simulink model "modelul2cerinta14"  (R2022b)
settings: Solver=VariableStepAuto  StartTime=0.0  StopTime=30  RelTol=1e-3
values from neighbouring files (symbols this model uses):
  SysLinD = c2d(SysLin,Te,'tustin')    [NeleptcuDanielAndrei.m]
  Te = 0.1    [NeleptcuDanielAndrei.m]
undefined symbols (not defined in the file or in its folder): par, ustar8, ystar8
settings Model: Creator=zuch3e  LastModifiedBy=zuch3e
settings DataIOCC: ReturnWorkspaceOutputs=off

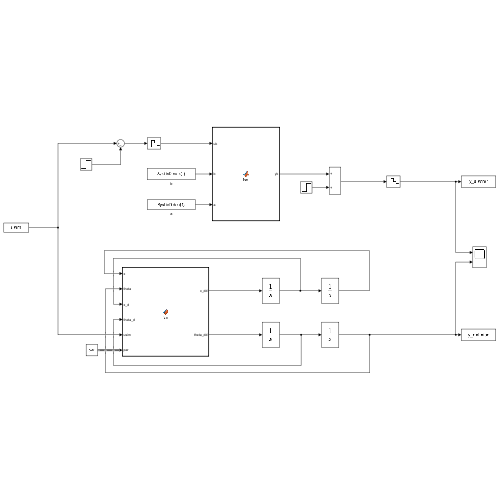
[thumbnail: Simulink's stored preview of the top-level diagram]
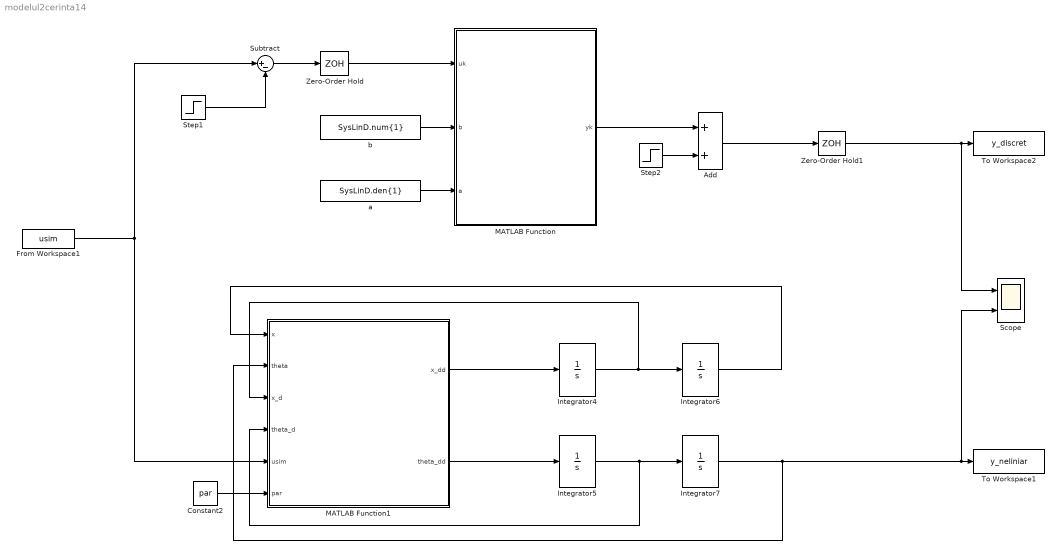
== system modelul2cerinta14 ==
  Add : Sum
  Constant2 : Constant  Value=par  OutDataTypeStr=Bus: par_bus
  From Workspace1 : FromWorkspace  VariableName=usim
  Integrator{4..7} (4 alike) : Integrator
  MATLAB Function : MATLAB Function  TreatAsAtomicUnit=on
  MATLAB Function1 : MATLAB Function  TreatAsAtomicUnit=on
  Scope : Scope  NumInputPorts=2
  Step1 : Step  After=ustar8  SampleTime=0
  Step2 : Step  After=ystar8  SampleTime=0
  Subtract : Sum  Inputs=|+-
  To Workspace1 : ToWorkspace  VariableName=y_neliniar  SaveFormat=Timeseries  SampleTime=-1
  To Workspace2 : ToWorkspace  VariableName=y_discret  SaveFormat=Timeseries  SampleTime=-1
  Zero-Order Hold : ZeroOrderHold  SampleTime=Te
  Zero-Order Hold1 : ZeroOrderHold  SampleTime=Te
  a : Constant  Value=SysLinD.den{1}
  b : Constant  Value=SysLinD.num{1}
  wires:
  Subtract/1 -> Zero-Order Hold/1
  Zero-Order Hold/1 -> MATLAB Function/1(uk)
  Add/1 -> Zero-Order Hold1/1
  Step1/1 -> Subtract/2
  Step2/1 -> Add/2
  From Workspace1/1 -> Subtract/1, MATLAB Function1/5(usim)
  b/1 -> MATLAB Function/2(b)
  a/1 -> MATLAB Function/3(a)
  Integrator4/1 -> MATLAB Function1/3(x_d), Integrator6/1
  Constant2/1 -> MATLAB Function1/6(par)
  Integrator5/1 -> MATLAB Function1/4(theta_d), Integrator7/1
  Integrator6/1 -> MATLAB Function1/1(x)
  MATLAB Function1/2(theta_dd) -> Integrator5/1
  Integrator7/1 -> MATLAB Function1/2(theta), Scope/2, To Workspace1/1
  MATLAB Function1/1(x_dd) -> Integrator4/1
  MATLAB Function/1(yk) -> Add/1
  Zero-Order Hold1/1 -> Scope/1, To Workspace2/1

== matlab function modelul2cerinta14/MATLAB Function1 ==
  data: x input; x_dd output; theta input; x_d input; theta_d input; usim input; par input; theta_dd output
function [x_dd, theta_dd] = fcn(x,theta,x_d,theta_d,usim, par)
x_dd = ((par.l0 + x) * (theta_d^2)) - (par.k*x)/par.m + par.g*cos(theta) - par.zeta*x_d;
theta_dd = ((-1)*par.g*sin(theta))/(par.l0 + x) - (2*x_d*theta_d)/(par.l0 + x) - par.zeta*theta_d + usim/(par.m*((par.l0 + x)^2));
end

== matlab function modelul2cerinta14/MATLAB Function ==
  data: uk input; yk output; b input; a input
function yk = fcn(uk,b,a)

persistent uk1 uk2 uk3 uk4 yk1 yk2 yk3 yk4

% b - coef pt numaratorul functiei de transfer
% a - coef pt numitorul functiei de transfer
[b0,b1,b2,b3,b4,a0,a1,a2,a3,a4] = deal(b(1),b(2),b(3),b(4),b(5),a(1),a(2),a(3),a(4),a(5));


%Verific daca sunt la inceput si nu am nimic in uk si yk
if isempty(uk1) && isempty(uk2) && isempty(uk3) && isempty(uk4) && isempty(yk1) && isempty(yk2) && isempty(yk3) && isempty(yk4)
    [uk1,uk2,uk3,uk4,yk1,yk2,yk3,yk4] = deal(0,0,0,0,0,0,0,0);
end


%Ecuatia cu diferente echivalenta cu cea construita in codul matlab
yk = (1/a0) * (b0*uk + b1*uk1 + b2*uk2 + b3*uk3 + b4*uk4 - a1*yk1 - a2*yk2 - a3*yk3 - a4*yk4);


%Updatare valori pentru pasul urmator
[uk1,uk2,uk3,uk4,yk1,yk2,yk3,yk4] = deal(uk,uk1,uk2,uk3,yk,yk1,yk2,yk3);

end
